simulink model "ProgrammingCalculator"  (R2017b)
settings: Solver=VariableStepAuto  StartTime=0.0  StopTime=10.0  RelTol=1e-3
settings Model: Creator=Hady Sallam  LastModifiedBy=Hady Sallam

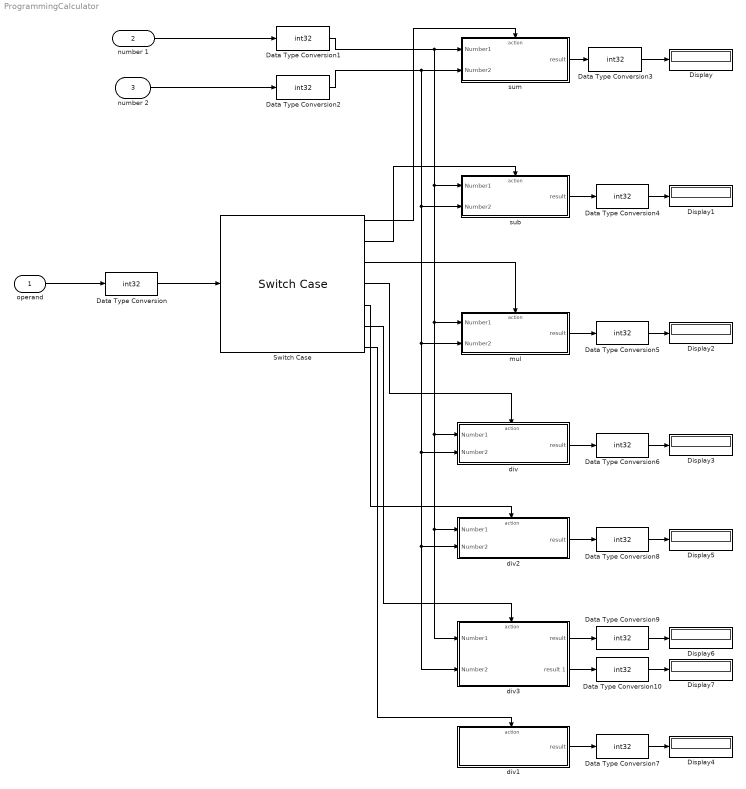
== system ProgrammingCalculator ==
  operand : Inport
  "number 1 " : Inport  Port=2
  number 2 : Inport  Port=3
  Data Type Conversion{,1..10} (11 alike) : DataTypeConversion  OutDataTypeStr=int32
  Display{,1..7} (8 alike) : Display
  Switch Case : SwitchCase  CaseConditions={1, 2, 3, 4 5 6}
  div : Subsystem  TreatAsAtomicUnit=on
  div1 : Subsystem  TreatAsAtomicUnit=on
  div2 : Subsystem  TreatAsAtomicUnit=on
  div3 : Subsystem  TreatAsAtomicUnit=on
  mul : Subsystem  TreatAsAtomicUnit=on
  sub : Subsystem  TreatAsAtomicUnit=on
  sum : Subsystem  TreatAsAtomicUnit=on
  wires:
  Data Type Conversion5/1 -> Display2/1
  div1/1("result ") -> Data Type Conversion7/1
  "number 1 "/1 -> Data Type Conversion1/1
  operand/1 -> Data Type Conversion/1
  sub/1(result) -> Data Type Conversion4/1
  Switch Case/3 -> mul/Action
  Data Type Conversion/1 -> Switch Case/1
  Data Type Conversion3/1 -> Display/1
  Data Type Conversion7/1 -> Display4/1
  number 2/1 -> Data Type Conversion2/1
  Switch Case/4 -> div/Action
  Switch Case/2 -> sub/Action
  div/1("result ") -> Data Type Conversion6/1
  sum/1("result ") -> Data Type Conversion3/1
  Switch Case/1 -> sum/Action
  Data Type Conversion6/1 -> Display3/1
  mul/1("result ") -> Data Type Conversion5/1
  Data Type Conversion4/1 -> Display1/1
  Switch Case/7 -> div1/Action
  div2/1("result ") -> Data Type Conversion8/1
  Data Type Conversion8/1 -> Display5/1
  Switch Case/5 -> div2/Action
  Switch Case/6 -> div3/Action
  Data Type Conversion9/1 -> Display6/1
  Data Type Conversion1/1 -> div3/1(Number1), div2/1(Number1), div/1(Number1), mul/1(Number1), sub/1(Number1), sum/1(Number1)
  Data Type Conversion2/1 -> div3/2(Number2), div2/2(Number2), div/2(Number2), mul/2(Number2), sub/2(Number2), sum/2(Number2)
  div3/1("result ") -> Data Type Conversion9/1
  div3/2(result 1) -> Data Type Conversion10/1
  Data Type Conversion10/1 -> Display7/1

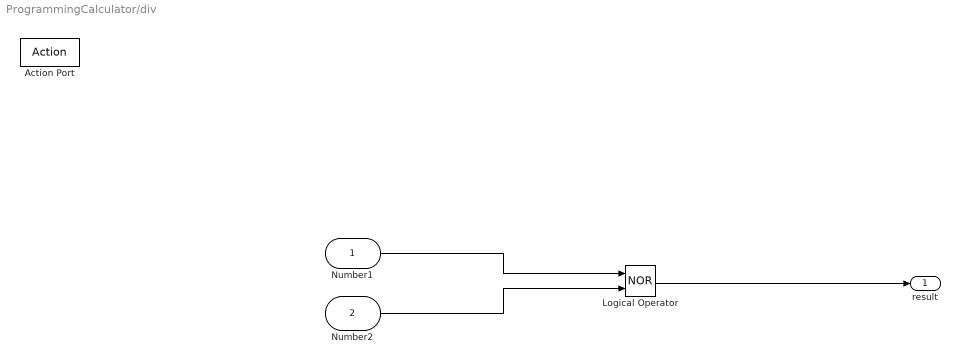
== system ProgrammingCalculator/div ==
  Number1 : Inport
  Number2 : Inport  Port=2
  Action Port : ActionPort  ActionType=case
  Logical Operator : Logic  Operator=NOR  AllPortsSameDT=off  OutDataTypeStr=boolean
  "result " : Outport
  wires:
  Logical Operator/1 -> "result "/1
  Number2/1 -> Logical Operator/2
  Number1/1 -> Logical Operator/1

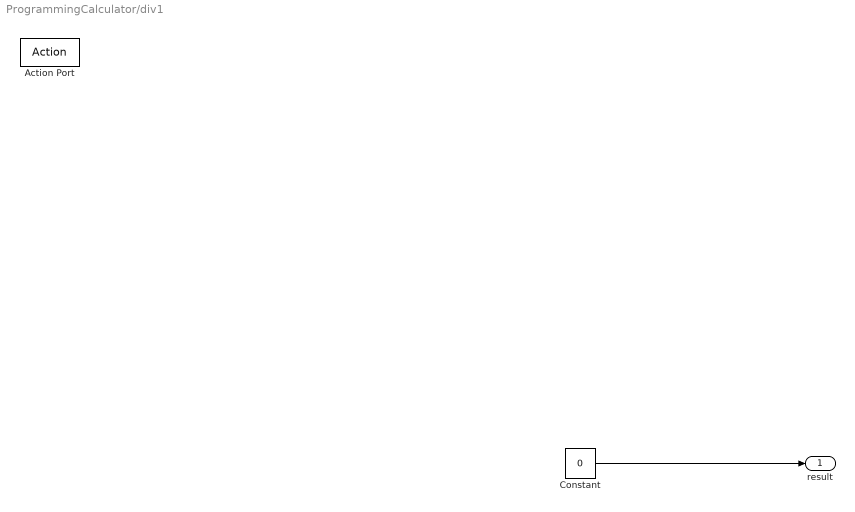
== system ProgrammingCalculator/div1 ==
  Action Port : ActionPort  ActionType=default
  Constant : Constant  Value=0
  "result " : Outport
  wires:
  Constant/1 -> "result "/1

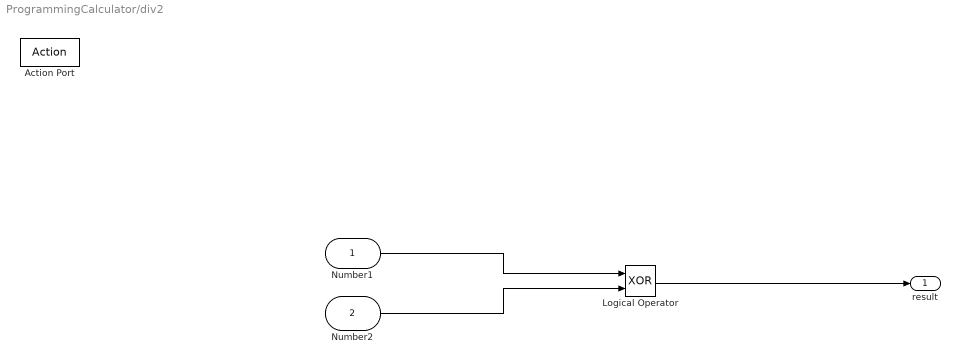
== system ProgrammingCalculator/div2 ==
  Number1 : Inport
  Number2 : Inport  Port=2
  Action Port : ActionPort  ActionType=case
  Logical Operator : Logic  Operator=XOR  AllPortsSameDT=off  OutDataTypeStr=boolean
  "result " : Outport
  wires:
  Logical Operator/1 -> "result "/1
  Number2/1 -> Logical Operator/2
  Number1/1 -> Logical Operator/1

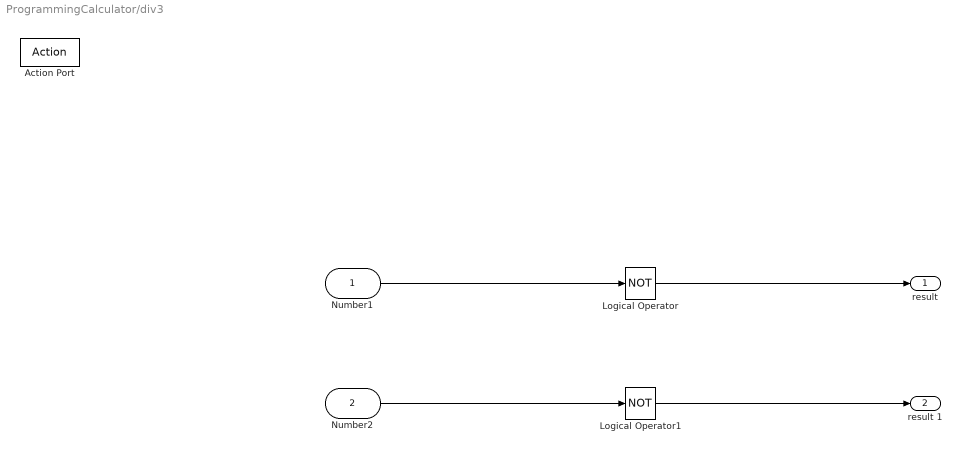
== system ProgrammingCalculator/div3 ==
  Number1 : Inport
  Number2 : Inport  Port=2
  Action Port : ActionPort  ActionType=case
  Logical Operator : Logic  Operator=NOT  AllPortsSameDT=off  OutDataTypeStr=boolean
  Logical Operator1 : Logic  Operator=NOT  AllPortsSameDT=off  OutDataTypeStr=boolean
  "result " : Outport
  result 1 : Outport  Port=2
  wires:
  Logical Operator/1 -> "result "/1
  Number1/1 -> Logical Operator/1
  Logical Operator1/1 -> result 1/1
  Number2/1 -> Logical Operator1/1

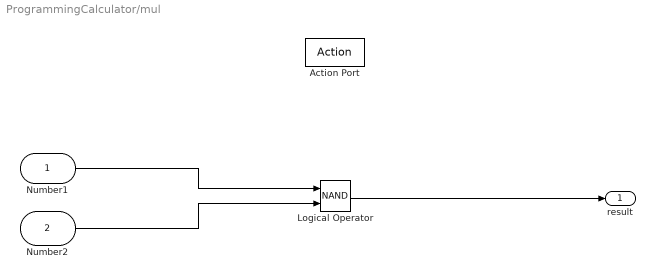
== system ProgrammingCalculator/mul ==
  Number1 : Inport
  Number2 : Inport  Port=2
  Action Port : ActionPort  ActionType=case
  Logical Operator : Logic  Operator=NAND  AllPortsSameDT=off  OutDataTypeStr=boolean
  "result " : Outport
  wires:
  Number1/1 -> Logical Operator/1
  Number2/1 -> Logical Operator/2
  Logical Operator/1 -> "result "/1

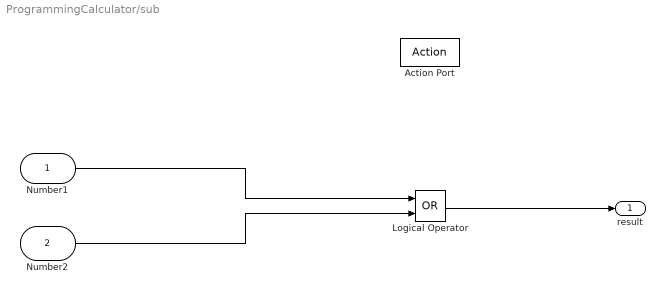
== system ProgrammingCalculator/sub ==
  Number1 : Inport
  Number2 : Inport  Port=2
  Action Port : ActionPort  ActionType=case
  Logical Operator : Logic  Operator=OR  AllPortsSameDT=off  OutDataTypeStr=boolean
  result : Outport
  wires:
  Number1/1 -> Logical Operator/1
  Number2/1 -> Logical Operator/2
  Logical Operator/1 -> result/1

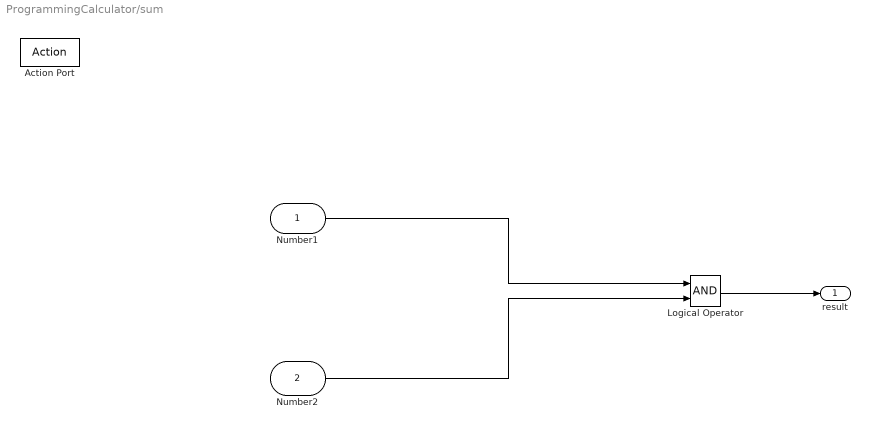
== system ProgrammingCalculator/sum ==
  Number1 : Inport
  Number2 : Inport  Port=2
  Action Port : ActionPort  ActionType=case
  Logical Operator : Logic  AllPortsSameDT=off  OutDataTypeStr=boolean
  "result " : Outport
  wires:
  Number2/1 -> Logical Operator/2
  Number1/1 -> Logical Operator/1
  Logical Operator/1 -> "result "/1
